simulink library "halin"  (R2021b)
settings: Solver=VariableStepAuto  StartTime=0.0  StopTime=10.0  RelTol=1e-3
undefined symbols (not defined in the file): TRUE
libraries: FVT_lib x177, hcu_lib x55
(part 8 of 17)

== system halin/HAL_IN/CAN3/BMS3 ==
  DT_CAN3_SG_BMS3 : Inport
  ACChrgCurrDis : Subsystem
  FireDetErr : Subsystem
  HVBChrgPwr : Subsystem
  HVBChrgPwrTotal : Subsystem
  HVBDrvPwr : Subsystem
  HVBDrvPwrTotal : Subsystem
  HVBFullChrgPwr : Subsystem
  HVBIsoImpedenceN : Subsystem
  HVBIsoImpedenceP : Subsystem
  HVBSOH : Subsystem
  HVBattErr : Subsystem
  HVBattPackVolt : Subsystem
  HVBattSOC : Subsystem
  HVBattSOCDis : Subsystem
  RemainChrgTime : Subsystem
  bus_selector : BusSelector  OutputSignals=CAN3_ACChrgCurrDis
  bus_selector1 : BusSelector  OutputSignals=CAN3_FireDetErr
  bus_selector10 : BusSelector  OutputSignals=CAN3_HVBattErr
  bus_selector11 : BusSelector  OutputSignals=CAN3_HVBattPackVolt
  bus_selector12 : BusSelector  OutputSignals=CAN3_HVBattSOC
  bus_selector13 : BusSelector  OutputSignals=CAN3_HVBattSOCDis
  bus_selector14 : BusSelector  OutputSignals=CAN3_RemainChrgTime
  bus_selector2 : BusSelector  OutputSignals=CAN3_HVBChrgPwr
  bus_selector3 : BusSelector  OutputSignals=CAN3_HVBChrgPwrTotal
  bus_selector4 : BusSelector  OutputSignals=CAN3_HVBDrvPwr
  bus_selector5 : BusSelector  OutputSignals=CAN3_HVBDrvPwrTotal
  bus_selector6 : BusSelector  OutputSignals=CAN3_HVBFullChrgPwr
  bus_selector7 : BusSelector  OutputSignals=CAN3_HVBIsoImpedenceN
  bus_selector8 : BusSelector  OutputSignals=CAN3_HVBIsoImpedenceP
  bus_selector9 : BusSelector  OutputSignals=CAN3_HVBSOH
  VHAL_ACChrgCurrDis_A : Outport
  VHAL_FireDetErr_flg : Outport  Port=2
  VHAL_HVBChrgPwr_kWh : Outport  Port=3
  VHAL_HVBChrgPwrTotal_kWh : Outport  Port=4
  VHAL_HVBDrvPwr_kWh : Outport  Port=5
  VHAL_HVBDrvPwrTotal_kWh : Outport  Port=6
  VHAL_HVBFullChrgPwr_kWh : Outport  Port=7
  VHAL_HVBIsoImpedenceN_Megaohm : Outport  Port=8
  VHAL_HVBIsoImpedenceP_Megaohm : Outport  Port=9
  VHAL_HVBSOH_pct : Outport  Port=10
  VHAL_HVBattErr_flg : Outport  Port=11
  VHAL_HVBattPackVolt_V : Outport  Port=12
  VHAL_HVBattSOC_pct : Outport  Port=13
  VHAL_HVBattSOCDis_pct : Outport  Port=14
  VHAL_RemainChrgTime_min : Outport  Port=15
  wires:
  DT_CAN3_SG_BMS3/1 -> [DT_CAN3_SG_BMS3]
  [DT_CAN3_SG_BMS3] -> bus_selector/1
  bus_selector/1 -> ACChrgCurrDis/1(ACChrgCurrDis)  "<CAN3_ACChrgCurrDis>"
  ACChrgCurrDis/1(VHAL_ACChrgCurrDis_A) -> VHAL_ACChrgCurrDis_A/1
  [DT_CAN3_SG_BMS3] -> bus_selector1/1
  bus_selector1/1 -> FireDetErr/1(FireDetErr)  "<CAN3_FireDetErr>"
  FireDetErr/1(VHAL_FireDetErr_flg) -> VHAL_FireDetErr_flg/1
  [DT_CAN3_SG_BMS3] -> bus_selector2/1
  bus_selector2/1 -> HVBChrgPwr/1(HVBChrgPwr)  "<CAN3_HVBChrgPwr>"
  HVBChrgPwr/1(VHAL_HVBChrgPwr_kWh) -> VHAL_HVBChrgPwr_kWh/1
  [DT_CAN3_SG_BMS3] -> bus_selector3/1
  bus_selector3/1 -> HVBChrgPwrTotal/1(HVBChrgPwrTotal)  "<CAN3_HVBChrgPwrTotal>"
  HVBChrgPwrTotal/1(VHAL_HVBChrgPwrTotal_kWh) -> VHAL_HVBChrgPwrTotal_kWh/1
  [DT_CAN3_SG_BMS3] -> bus_selector4/1
  bus_selector4/1 -> HVBDrvPwr/1(HVBDrvPwr)  "<CAN3_HVBDrvPwr>"
  HVBDrvPwr/1(VHAL_HVBDrvPwr_kWh) -> VHAL_HVBDrvPwr_kWh/1
  [DT_CAN3_SG_BMS3] -> bus_selector5/1
  bus_selector5/1 -> HVBDrvPwrTotal/1(HVBDrvPwrTotal)  "<CAN3_HVBDrvPwrTotal>"
  HVBDrvPwrTotal/1(VHAL_HVBDrvPwrTotal_kWh) -> VHAL_HVBDrvPwrTotal_kWh/1
  [DT_CAN3_SG_BMS3] -> bus_selector6/1
  bus_selector6/1 -> HVBFullChrgPwr/1(HVBFullChrgPwr)  "<CAN3_HVBFullChrgPwr>"
  HVBFullChrgPwr/1(VHAL_HVBFullChrgPwr_kWh) -> VHAL_HVBFullChrgPwr_kWh/1
  [DT_CAN3_SG_BMS3] -> bus_selector7/1
  bus_selector7/1 -> HVBIsoImpedenceN/1(HVBIsoImpedenceN)  "<CAN3_HVBIsoImpedenceN>"
  HVBIsoImpedenceN/1(VHAL_HVBIsoImpedenceN_Megaohm) -> VHAL_HVBIsoImpedenceN_Megaohm/1
  [DT_CAN3_SG_BMS3] -> bus_selector8/1
  bus_selector8/1 -> HVBIsoImpedenceP/1(HVBIsoImpedenceP)  "<CAN3_HVBIsoImpedenceP>"
  HVBIsoImpedenceP/1(VHAL_HVBIsoImpedenceP_Megaohm) -> VHAL_HVBIsoImpedenceP_Megaohm/1
  [DT_CAN3_SG_BMS3] -> bus_selector9/1
  bus_selector9/1 -> HVBSOH/1(HVBSOH)  "<CAN3_HVBSOH>"
  HVBSOH/1(VHAL_HVBSOH_pct) -> VHAL_HVBSOH_pct/1
  [DT_CAN3_SG_BMS3] -> bus_selector10/1
  bus_selector10/1 -> HVBattErr/1(HVBattErr)  "<CAN3_HVBattErr>"
  HVBattErr/1(VHAL_HVBattErr_flg) -> VHAL_HVBattErr_flg/1
  [DT_CAN3_SG_BMS3] -> bus_selector11/1
  bus_selector11/1 -> HVBattPackVolt/1(HVBattPackVolt)  "<CAN3_HVBattPackVolt>"
  HVBattPackVolt/1(VHAL_HVBattPackVolt_V) -> VHAL_HVBattPackVolt_V/1
  [DT_CAN3_SG_BMS3] -> bus_selector12/1
  bus_selector12/1 -> HVBattSOC/1(HVBattSOC)  "<CAN3_HVBattSOC>"
  HVBattSOC/1(VHAL_HVBattSOC_pct) -> VHAL_HVBattSOC_pct/1
  [DT_CAN3_SG_BMS3] -> bus_selector13/1
  bus_selector13/1 -> HVBattSOCDis/1(HVBattSOCDis)  "<CAN3_HVBattSOCDis>"
  HVBattSOCDis/1(VHAL_HVBattSOCDis_pct) -> VHAL_HVBattSOCDis_pct/1
  [DT_CAN3_SG_BMS3] -> bus_selector14/1
  bus_selector14/1 -> RemainChrgTime/1(RemainChrgTime)  "<CAN3_RemainChrgTime>"
  RemainChrgTime/1(VHAL_RemainChrgTime_min) -> VHAL_RemainChrgTime_min/1

== system halin/HAL_IN/CAN3/BMS4 ==
  DT_CAN3_SG_BMS4 : Inport
  CellTempAvg : Subsystem
  HVBCellVoltMax : Subsystem
  HVBCellVoltMin : Subsystem
  HVBMTempMax : Subsystem
  HVBMTempMin : Subsystem
  MaxCellTempNum : Subsystem
  MaxCellVoltNum : Subsystem
  MinCellTempNum : Subsystem
  MinCellVoltNum : Subsystem
  bus_selector : BusSelector  OutputSignals=CAN3_CellTempAvg
  bus_selector1 : BusSelector  OutputSignals=CAN3_HVBCellVoltMax
  bus_selector2 : BusSelector  OutputSignals=CAN3_HVBCellVoltMin
  bus_selector3 : BusSelector  OutputSignals=CAN3_HVBMTempMax
  bus_selector4 : BusSelector  OutputSignals=CAN3_HVBMTempMin
  bus_selector5 : BusSelector  OutputSignals=CAN3_MaxCellTemp_Num
  bus_selector6 : BusSelector  OutputSignals=CAN3_MaxCellVolt_Num
  bus_selector7 : BusSelector  OutputSignals=CAN3_MinCellTemp_Num
  bus_selector8 : BusSelector  OutputSignals=CAN3_MinCellVolt_Num
  VHAL_CellTempAvg_C : Outport
  VHAL_HVBCellVoltMax_mV : Outport  Port=2
  VHAL_HVBCellVoltMin_mV : Outport  Port=3
  VHAL_HVBMTempMax_C : Outport  Port=4
  VHAL_HVBMTempMin_C : Outport  Port=5
  VHAL_MaxCellTempNum_enum : Outport  Port=6
  VHAL_MaxCellVoltNum_enum : Outport  Port=7
  VHAL_MinCellTempNum_enum : Outport  Port=8
  VHAL_MinCellVoltNum_enum : Outport  Port=9
  wires:
  DT_CAN3_SG_BMS4/1 -> [DT_CAN3_SG_BMS4]
  [DT_CAN3_SG_BMS4] -> bus_selector/1
  bus_selector/1 -> CellTempAvg/1(CellTempAvg)  "<CAN3_CellTempAvg>"
  CellTempAvg/1(VHAL_CellTempAvg_C) -> VHAL_CellTempAvg_C/1
  [DT_CAN3_SG_BMS4] -> bus_selector1/1
  bus_selector1/1 -> HVBCellVoltMax/1(HVBCellVoltMax)  "<CAN3_HVBCellVoltMax>"
  HVBCellVoltMax/1(VHAL_HVBCellVoltMax_mV) -> VHAL_HVBCellVoltMax_mV/1
  [DT_CAN3_SG_BMS4] -> bus_selector2/1
  bus_selector2/1 -> HVBCellVoltMin/1(HVBCellVoltMin)  "<CAN3_HVBCellVoltMin>"
  HVBCellVoltMin/1(VHAL_HVBCellVoltMin_mV) -> VHAL_HVBCellVoltMin_mV/1
  [DT_CAN3_SG_BMS4] -> bus_selector3/1
  bus_selector3/1 -> HVBMTempMax/1(HVBMTempMax)  "<CAN3_HVBMTempMax>"
  HVBMTempMax/1(VHAL_HVBMTempMax_C) -> VHAL_HVBMTempMax_C/1
  [DT_CAN3_SG_BMS4] -> bus_selector4/1
  bus_selector4/1 -> HVBMTempMin/1(HVBMTempMin)  "<CAN3_HVBMTempMin>"
  HVBMTempMin/1(VHAL_HVBMTempMin_C) -> VHAL_HVBMTempMin_C/1
  [DT_CAN3_SG_BMS4] -> bus_selector5/1
  bus_selector5/1 -> MaxCellTempNum/1(MaxCellTemp_Num)  "<CAN3_MaxCellTemp_Num>"
  MaxCellTempNum/1(VHAL_MaxCellTempNum_enum) -> VHAL_MaxCellTempNum_enum/1
  [DT_CAN3_SG_BMS4] -> bus_selector6/1
  bus_selector6/1 -> MaxCellVoltNum/1(MaxCellVolt_Num)  "<CAN3_MaxCellVolt_Num>"
  MaxCellVoltNum/1(VHAL_MaxCellVoltNum_enum) -> VHAL_MaxCellVoltNum_enum/1
  [DT_CAN3_SG_BMS4] -> bus_selector7/1
  bus_selector7/1 -> MinCellTempNum/1(MinCellTemp_Num)  "<CAN3_MinCellTemp_Num>"
  MinCellTempNum/1(VHAL_MinCellTempNum_enum) -> VHAL_MinCellTempNum_enum/1
  [DT_CAN3_SG_BMS4] -> bus_selector8/1
  bus_selector8/1 -> MinCellVoltNum/1(MinCellVolt_Num)  "<CAN3_MinCellVolt_Num>"
  MinCellVoltNum/1(VHAL_MinCellVoltNum_enum) -> VHAL_MinCellVoltNum_enum/1

== system halin/HAL_IN/CAN3/BMS5 ==
  DT_CAN3_SG_BMS5 : Inport
  HVInVolt : Subsystem
  LVBattDet12V : Subsystem
  OBCACCSLimit : Subsystem
  OBCDCCurLm : Subsystem
  OBCDCVoltLm : Subsystem
  bus_selector : BusSelector  OutputSignals=CAN3_HVInVolt
  bus_selector1 : BusSelector  OutputSignals=CAN3_LVBattDet12V
  bus_selector2 : BusSelector  OutputSignals=CAN3_OBCACCSLimit
  bus_selector3 : BusSelector  OutputSignals=CAN3_OBCDCCurLm
  bus_selector4 : BusSelector  OutputSignals=CAN3_OBCDCVoltLm
  VHAL_HVInVolt_V : Outport
  VHAL_LVBattDet12V_V : Outport  Port=2
  VHAL_OBCACCSLimit_A : Outport  Port=3
  VHAL_OBCDCCurLm_A : Outport  Port=4
  VHAL_OBCDCVoltLm_V : Outport  Port=5
  wires:
  DT_CAN3_SG_BMS5/1 -> [DT_CAN3_SG_BMS5]
  [DT_CAN3_SG_BMS5] -> bus_selector/1
  bus_selector/1 -> HVInVolt/1(HVInVolt)  "<CAN3_HVInVolt>"
  HVInVolt/1(VHAL_HVInVolt_V) -> VHAL_HVInVolt_V/1
  [DT_CAN3_SG_BMS5] -> bus_selector1/1
  bus_selector1/1 -> LVBattDet12V/1(LVBattDet12V)  "<CAN3_LVBattDet12V>"
  LVBattDet12V/1(VHAL_LVBattDet12V_V) -> VHAL_LVBattDet12V_V/1
  [DT_CAN3_SG_BMS5] -> bus_selector2/1
  bus_selector2/1 -> OBCACCSLimit/1(OBCACCSLimit)  "<CAN3_OBCACCSLimit>"
  OBCACCSLimit/1(VHAL_OBCACCSLimit_A) -> VHAL_OBCACCSLimit_A/1
  [DT_CAN3_SG_BMS5] -> bus_selector3/1
  bus_selector3/1 -> OBCDCCurLm/1(OBCDCCurLm)  "<CAN3_OBCDCCurLm>"
  OBCDCCurLm/1(VHAL_OBCDCCurLm_A) -> VHAL_OBCDCCurLm_A/1
  [DT_CAN3_SG_BMS5] -> bus_selector4/1
  bus_selector4/1 -> OBCDCVoltLm/1(OBCDCVoltLm)  "<CAN3_OBCDCVoltLm>"
  OBCDCVoltLm/1(VHAL_OBCDCVoltLm_V) -> VHAL_OBCDCVoltLm_V/1

== system halin/HAL_IN/CAN3/BMS6 ==
  DT_CAN3_SG_BMS6 : Inport
  BMSChckSum : Subsystem
  BMSREADY : Subsystem
  BMSRolCnct : Subsystem
  BMSWarn1 : Subsystem
  BMSWarn2 : Subsystem
  BMSWarn3 : Subsystem
  BMSWarn4 : Subsystem
  BMSWarn5 : Subsystem
  BMSWarn6 : Subsystem
  BMSWarn7 : Subsystem
  BMSWarn8 : Subsystem
  ChrgInLockReq : Subsystem
  ChrgPlugSta : Subsystem
  DisChrgPlugErr : Subsystem
  ExtChrgSta : Subsystem
  HVBChrgErr : Subsystem
  HVBContactorSta : Subsystem
  HVBHVILErr : Subsystem
  HVBOvrTempErr : Subsystem
  HVBOvrTempWarn : Subsystem
  HVBPreheatPrecoolSta : Subsystem
  HVBattReady4Pre : Subsystem
  HVILSta : Subsystem
  V2LSta : Subsystem
  bus_selector : BusSelector  OutputSignals=CAN3_BMSChckSum
  bus_selector1 : BusSelector  OutputSignals=CAN3_BMSRolCnct
  bus_selector10 : BusSelector  OutputSignals=CAN3_BMS_Warn_8
  bus_selector11 : BusSelector  OutputSignals=CAN3_ChrgInLockReq
  bus_selector12 : BusSelector  OutputSignals=CAN3_ChrgPlugSta
  bus_selector13 : BusSelector  OutputSignals=CAN3_DisChrgPlugErr
  bus_selector14 : BusSelector  OutputSignals=CAN3_ExtChrgSta
  bus_selector15 : BusSelector  OutputSignals=CAN3_HVBChrgErr
  bus_selector16 : BusSelector  OutputSignals=CAN3_HVBContactorSta
  bus_selector17 : BusSelector  OutputSignals=CAN3_HVBHVILErr
  bus_selector18 : BusSelector  OutputSignals=CAN3_HVBOvrTempErr
  bus_selector19 : BusSelector  OutputSignals=CAN3_HVBOvrTempWarn
  bus_selector2 : BusSelector  OutputSignals=CAN3_BMS_READY
  bus_selector20 : BusSelector  OutputSignals=CAN3_HVBPreheatPrecoolSta
  bus_selector21 : BusSelector  OutputSignals=CAN3_HVBattReady4Pre
  bus_selector22 : BusSelector  OutputSignals=CAN3_HVILSta
  bus_selector23 : BusSelector  OutputSignals=CAN3_V2LSta
  bus_selector3 : BusSelector  OutputSignals=CAN3_BMS_Warn_1
  bus_selector4 : BusSelector  OutputSignals=CAN3_BMS_Warn_2
  bus_selector5 : BusSelector  OutputSignals=CAN3_BMS_Warn_3
  bus_selector6 : BusSelector  OutputSignals=CAN3_BMS_Warn_4
  bus_selector7 : BusSelector  OutputSignals=CAN3_BMS_Warn_5
  bus_selector8 : BusSelector  OutputSignals=CAN3_BMS_Warn_6
  bus_selector9 : BusSelector  OutputSignals=CAN3_BMS_Warn_7
  VHAL_BMSChckSum_enum : Outport
  VHAL_BMSRolCnct_enum : Outport  Port=2
  VHAL_BMSREADY_flg : Outport  Port=3
  VHAL_BMSWarn1_flg : Outport  Port=4
  VHAL_BMSWarn2_flg : Outport  Port=5
  VHAL_BMSWarn3_flg : Outport  Port=6
  VHAL_BMSWarn4_flg : Outport  Port=7
  VHAL_BMSWarn5_flg : Outport  Port=8
  VHAL_BMSWarn6_flg : Outport  Port=9
  VHAL_BMSWarn7_flg : Outport  Port=10
  VHAL_BMSWarn8_flg : Outport  Port=11
  VHAL_ChrgInLockReq_enum : Outport  Port=12
  VHAL_ChrgPlugSta_enum : Outport  Port=13
  VHAL_DisChrgPlugErr_enum : Outport  Port=14
  VHAL_ExtChrgSta_enum : Outport  Port=15
  VHAL_HVBChrgErr_enum : Outport  Port=16
  VHAL_HVBContactorSta_flg : Outport  Port=17
  VHAL_HVBHVILErr_flg : Outport  Port=18
  VHAL_HVBOvrTempErr_flg : Outport  Port=19
  VHAL_HVBOvrTempWarn_enum : Outport  Port=20
  VHAL_HVBPreheatPrecoolSta_enum : Outport  Port=21
  VHAL_HVBattReady4Pre_enum : Outport  Port=22
  VHAL_HVILSta_flg : Outport  Port=23
  VHAL_V2LSta_enum : Outport  Port=24
  wires:
  DT_CAN3_SG_BMS6/1 -> [DT_CAN3_SG_BMS6]
  [DT_CAN3_SG_BMS6] -> bus_selector/1
  bus_selector/1 -> BMSChckSum/1(BMSChckSum)  "<CAN3_BMSChckSum>"
  BMSChckSum/1(VHAL_BMSChckSum_enum) -> VHAL_BMSChckSum_enum/1
  [DT_CAN3_SG_BMS6] -> bus_selector1/1
  bus_selector1/1 -> BMSRolCnct/1(BMSRolCnct)  "<CAN3_BMSRolCnct>"
  BMSRolCnct/1(VHAL_BMSRolCnct_enum) -> VHAL_BMSRolCnct_enum/1
  [DT_CAN3_SG_BMS6] -> bus_selector2/1
  bus_selector2/1 -> BMSREADY/1(BMS_READY)  "<CAN3_BMS_READY>"
  BMSREADY/1(VHAL_BMSREADY_flg) -> VHAL_BMSREADY_flg/1
  [DT_CAN3_SG_BMS6] -> bus_selector3/1
  bus_selector3/1 -> BMSWarn1/1(BMS_Warn_1)  "<CAN3_BMS_Warn_1>"
  BMSWarn1/1(VHAL_BMSWarn1_flg) -> VHAL_BMSWarn1_flg/1
  [DT_CAN3_SG_BMS6] -> bus_selector4/1
  bus_selector4/1 -> BMSWarn2/1(BMS_Warn_2)  "<CAN3_BMS_Warn_2>"
  BMSWarn2/1(VHAL_BMSWarn2_flg) -> VHAL_BMSWarn2_flg/1
  [DT_CAN3_SG_BMS6] -> bus_selector5/1
  bus_selector5/1 -> BMSWarn3/1(BMS_Warn_3)  "<CAN3_BMS_Warn_3>"
  BMSWarn3/1(VHAL_BMSWarn3_flg) -> VHAL_BMSWarn3_flg/1
  [DT_CAN3_SG_BMS6] -> bus_selector6/1
  bus_selector6/1 -> BMSWarn4/1(BMS_Warn_4)  "<CAN3_BMS_Warn_4>"
  BMSWarn4/1(VHAL_BMSWarn4_flg) -> VHAL_BMSWarn4_flg/1
  [DT_CAN3_SG_BMS6] -> bus_selector7/1
  bus_selector7/1 -> BMSWarn5/1(BMS_Warn_5)  "<CAN3_BMS_Warn_5>"
  BMSWarn5/1(VHAL_BMSWarn5_flg) -> VHAL_BMSWarn5_flg/1
  [DT_CAN3_SG_BMS6] -> bus_selector8/1
  bus_selector8/1 -> BMSWarn6/1(BMS_Warn_6)  "<CAN3_BMS_Warn_6>"
  BMSWarn6/1(VHAL_BMSWarn6_flg) -> VHAL_BMSWarn6_flg/1
  [DT_CAN3_SG_BMS6] -> bus_selector9/1
  bus_selector9/1 -> BMSWarn7/1(BMS_Warn_7)  "<CAN3_BMS_Warn_7>"
  BMSWarn7/1(VHAL_BMSWarn7_flg) -> VHAL_BMSWarn7_flg/1
  [DT_CAN3_SG_BMS6] -> bus_selector10/1
  bus_selector10/1 -> BMSWarn8/1(BMS_Warn_8)  "<CAN3_BMS_Warn_8>"
  BMSWarn8/1(VHAL_BMSWarn8_flg) -> VHAL_BMSWarn8_flg/1
  [DT_CAN3_SG_BMS6] -> bus_selector11/1
  bus_selector11/1 -> ChrgInLockReq/1(ChrgInLockReq)  "<CAN3_ChrgInLockReq>"
  ChrgInLockReq/1(VHAL_ChrgInLockReq_enum) -> VHAL_ChrgInLockReq_enum/1
  [DT_CAN3_SG_BMS6] -> bus_selector12/1
  bus_selector12/1 -> ChrgPlugSta/1(ChrgPlugSta)  "<CAN3_ChrgPlugSta>"
  ChrgPlugSta/1(VHAL_ChrgPlugSta_enum) -> VHAL_ChrgPlugSta_enum/1
  [DT_CAN3_SG_BMS6] -> bus_selector13/1
  bus_selector13/1 -> DisChrgPlugErr/1(DisChrgPlugErr)  "<CAN3_DisChrgPlugErr>"
  DisChrgPlugErr/1(VHAL_DisChrgPlugErr_enum) -> VHAL_DisChrgPlugErr_enum/1
  [DT_CAN3_SG_BMS6] -> bus_selector14/1
  bus_selector14/1 -> ExtChrgSta/1(ExtChrgSta)  "<CAN3_ExtChrgSta>"
  ExtChrgSta/1(VHAL_ExtChrgSta_enum) -> VHAL_ExtChrgSta_enum/1
  [DT_CAN3_SG_BMS6] -> bus_selector15/1
  bus_selector15/1 -> HVBChrgErr/1(HVBChrgErr)  "<CAN3_HVBChrgErr>"
  HVBChrgErr/1(VHAL_HVBChrgErr_enum) -> VHAL_HVBChrgErr_enum/1
  [DT_CAN3_SG_BMS6] -> bus_selector16/1
  bus_selector16/1 -> HVBContactorSta/1(HVBContactorSta)  "<CAN3_HVBContactorSta>"
  HVBContactorSta/1(VHAL_HVBContactorSta_flg) -> VHAL_HVBContactorSta_flg/1
  [DT_CAN3_SG_BMS6] -> bus_selector17/1
  bus_selector17/1 -> HVBHVILErr/1(HVBHVILErr)  "<CAN3_HVBHVILErr>"
  HVBHVILErr/1(VHAL_HVBHVILErr_flg) -> VHAL_HVBHVILErr_flg/1
  [DT_CAN3_SG_BMS6] -> bus_selector18/1
  bus_selector18/1 -> HVBOvrTempErr/1(HVBOvrTempErr)  "<CAN3_HVBOvrTempErr>"
  HVBOvrTempErr/1(VHAL_HVBOvrTempErr_flg) -> VHAL_HVBOvrTempErr_flg/1
  [DT_CAN3_SG_BMS6] -> bus_selector19/1
  bus_selector19/1 -> HVBOvrTempWarn/1(HVBOvrTempWarn)  "<CAN3_HVBOvrTempWarn>"
  HVBOvrTempWarn/1(VHAL_HVBOvrTempWarn_enum) -> VHAL_HVBOvrTempWarn_enum/1
  [DT_CAN3_SG_BMS6] -> bus_selector20/1
  bus_selector20/1 -> HVBPreheatPrecoolSta/1(HVBPreheatPrecoolSta)  "<CAN3_HVBPreheatPrecoolSta>"
  HVBPreheatPrecoolSta/1(VHAL_HVBPreheatPrecoolSta_enum) -> VHAL_HVBPreheatPrecoolSta_enum/1
  [DT_CAN3_SG_BMS6] -> bus_selector21/1
  bus_selector21/1 -> HVBattReady4Pre/1(HVBattReady4Pre)  "<CAN3_HVBattReady4Pre>"
  HVBattReady4Pre/1(VHAL_HVBattReady4Pre_enum) -> VHAL_HVBattReady4Pre_enum/1
  [DT_CAN3_SG_BMS6] -> bus_selector22/1
  bus_selector22/1 -> HVILSta/1(HVILSta)  "<CAN3_HVILSta>"
  HVILSta/1(VHAL_HVILSta_flg) -> VHAL_HVILSta_flg/1
  [DT_CAN3_SG_BMS6] -> bus_selector23/1
  bus_selector23/1 -> V2LSta/1(V2LSta)  "<CAN3_V2LSta>"
  V2LSta/1(VHAL_V2LSta_enum) -> VHAL_V2LSta_enum/1

== system halin/HAL_IN/CAN3/BMS8 ==
  DT_CAN3_SG_BMS8 : Inport
  MainRlyNegSta : Subsystem
  MainRlyPosSta : Subsystem
  bus_selector : BusSelector  OutputSignals=CAN3_MainRlyNegSta
  bus_selector1 : BusSelector  OutputSignals=CAN3_MainRlyPosSta
  VHAL_MainRlyNegSta_enum : Outport
  VHAL_MainRlyPosSta_enum : Outport  Port=2
  wires:
  DT_CAN3_SG_BMS8/1 -> [DT_CAN3_SG_BMS8]
  [DT_CAN3_SG_BMS8] -> bus_selector/1
  bus_selector/1 -> MainRlyNegSta/1(MainRlyNegSta)  "<CAN3_MainRlyNegSta>"
  MainRlyNegSta/1(VHAL_MainRlyNegSta_enum) -> VHAL_MainRlyNegSta_enum/1
  [DT_CAN3_SG_BMS8] -> bus_selector1/1
  bus_selector1/1 -> MainRlyPosSta/1(MainRlyPosSta)  "<CAN3_MainRlyPosSta>"
  MainRlyPosSta/1(VHAL_MainRlyPosSta_enum) -> VHAL_MainRlyPosSta_enum/1

== system halin/HAL_IN/CAN3/CCU1 ==
  DT_CAN3_SG_CCU1 : Inport
  CSCCU1 : Subsystem
  DCDCAuxCur : Subsystem
  DCDCAuxVolt : Subsystem
  DCDCHVCur : Subsystem
  DCDCInVoltInf : Subsystem
  DCDCPreCompleted : Subsystem
  OBCDCCurrInf : Subsystem
  OBCDCVoltInf : Subsystem
  OBCPreCompleted : Subsystem
  OBCWakeup4Plugin : Subsystem
  RCCCU1 : Subsystem
  bus_selector : BusSelector  OutputSignals=CAN3_CS_CCU1
  bus_selector1 : BusSelector  OutputSignals=CAN3_DCDCAuxCur
  bus_selector10 : BusSelector  OutputSignals=CAN3_RC_CCU1
  bus_selector2 : BusSelector  OutputSignals=CAN3_DCDCAuxVolt
  bus_selector3 : BusSelector  OutputSignals=CAN3_DCDCHVCur
  bus_selector4 : BusSelector  OutputSignals=CAN3_DCDCInVoltInf
  bus_selector5 : BusSelector  OutputSignals=CAN3_DCDCPreCompleted
  bus_selector6 : BusSelector  OutputSignals=CAN3_OBCDCCurrInf
  bus_selector7 : BusSelector  OutputSignals=CAN3_OBCDCVoltInf
  bus_selector8 : BusSelector  OutputSignals=CAN3_OBCPreCompleted
  bus_selector9 : BusSelector  OutputSignals=CAN3_OBCWakeup4Plugin
  VHAL_CSCCU1_enum : Outport
  VHAL_DCDCAuxCur_A : Outport  Port=2
  VHAL_DCDCAuxVolt_V : Outport  Port=3
  VHAL_DCDCHVCur_A : Outport  Port=4
  VHAL_DCDCInVoltInf_V : Outport  Port=5
  VHAL_DCDCPreCompleted_enum : Outport  Port=6
  VHAL_OBCDCCurrInf_A : Outport  Port=7
  VHAL_OBCDCVoltInf_V : Outport  Port=8
  VHAL_OBCPreCompleted_enum : Outport  Port=9
  VHAL_OBCWakeup4Plugin_flg : Outport  Port=10
  VHAL_RCCCU1_enum : Outport  Port=11
  wires:
  DT_CAN3_SG_CCU1/1 -> [DT_CAN3_SG_CCU1]
  [DT_CAN3_SG_CCU1] -> bus_selector/1
  bus_selector/1 -> CSCCU1/1(CS_CCU1)  "<CAN3_CS_CCU1>"
  CSCCU1/1(VHAL_CSCCU1_enum) -> VHAL_CSCCU1_enum/1
  [DT_CAN3_SG_CCU1] -> bus_selector1/1
  bus_selector1/1 -> DCDCAuxCur/1(DCDCAuxCur)  "<CAN3_DCDCAuxCur>"
  DCDCAuxCur/1(VHAL_DCDCAuxCur_A) -> VHAL_DCDCAuxCur_A/1
  [DT_CAN3_SG_CCU1] -> bus_selector2/1
  bus_selector2/1 -> DCDCAuxVolt/1(DCDCAuxVolt)  "<CAN3_DCDCAuxVolt>"
  DCDCAuxVolt/1(VHAL_DCDCAuxVolt_V) -> VHAL_DCDCAuxVolt_V/1
  [DT_CAN3_SG_CCU1] -> bus_selector3/1
  bus_selector3/1 -> DCDCHVCur/1(DCDCHVCur)  "<CAN3_DCDCHVCur>"
  DCDCHVCur/1(VHAL_DCDCHVCur_A) -> VHAL_DCDCHVCur_A/1
  [DT_CAN3_SG_CCU1] -> bus_selector4/1
  bus_selector4/1 -> DCDCInVoltInf/1(DCDCInVoltInf)  "<CAN3_DCDCInVoltInf>"
  DCDCInVoltInf/1(VHAL_DCDCInVoltInf_V) -> VHAL_DCDCInVoltInf_V/1
  [DT_CAN3_SG_CCU1] -> bus_selector5/1
  bus_selector5/1 -> DCDCPreCompleted/1(DCDCPreCompleted)  "<CAN3_DCDCPreCompleted>"
  DCDCPreCompleted/1(VHAL_DCDCPreCompleted_enum) -> VHAL_DCDCPreCompleted_enum/1
  [DT_CAN3_SG_CCU1] -> bus_selector6/1
  bus_selector6/1 -> OBCDCCurrInf/1(OBCDCCurrInf)  "<CAN3_OBCDCCurrInf>"
  OBCDCCurrInf/1(VHAL_OBCDCCurrInf_A) -> VHAL_OBCDCCurrInf_A/1
  [DT_CAN3_SG_CCU1] -> bus_selector7/1
  bus_selector7/1 -> OBCDCVoltInf/1(OBCDCVoltInf)  "<CAN3_OBCDCVoltInf>"
  OBCDCVoltInf/1(VHAL_OBCDCVoltInf_V) -> VHAL_OBCDCVoltInf_V/1
  [DT_CAN3_SG_CCU1] -> bus_selector8/1
  bus_selector8/1 -> OBCPreCompleted/1(OBCPreCompleted)  "<CAN3_OBCPreCompleted>"
  OBCPreCompleted/1(VHAL_OBCPreCompleted_enum) -> VHAL_OBCPreCompleted_enum/1
  [DT_CAN3_SG_CCU1] -> bus_selector9/1
  bus_selector9/1 -> OBCWakeup4Plugin/1(OBCWakeup4Plugin)  "<CAN3_OBCWakeup4Plugin>"
  OBCWakeup4Plugin/1(VHAL_OBCWakeup4Plugin_flg) -> VHAL_OBCWakeup4Plugin_flg/1
  [DT_CAN3_SG_CCU1] -> bus_selector10/1
  bus_selector10/1 -> RCCCU1/1(RC_CCU1)  "<CAN3_RC_CCU1>"
  RCCCU1/1(VHAL_RCCCU1_enum) -> VHAL_RCCCU1_enum/1

== system halin/HAL_IN/CAN3/CCU2 ==
  DT_CAN3_SG_CCU2 : Inport
  CSCCU2 : Subsystem
  DCDCEnaSta : Subsystem
  DCDCFaultSta : Subsystem
  DCDCReady4Pre : Subsystem
  DCDCTemp : Subsystem
  OBCACCurLim : Subsystem
  OBCACCurrInf : Subsystem
  OBCACVoltInf : Subsystem
  OBCEnaSta : Subsystem
  OBCFaultSta : Subsystem
  OBCPluginSta : Subsystem
  OBCReady4Pre : Subsystem
  OBCTemp : Subsystem
  OBCV2LSta : Subsystem
  RCCCU2 : Subsystem
  bus_selector : BusSelector  OutputSignals=CAN3_CS_CCU2
  bus_selector1 : BusSelector  OutputSignals=CAN3_DCDCEnaSta
  bus_selector10 : BusSelector  OutputSignals=CAN3_OBCReady4Pre
  bus_selector11 : BusSelector  OutputSignals=CAN3_OBCTemp
  bus_selector12 : BusSelector  OutputSignals=CAN3_OBCV2LSta
  bus_selector13 : BusSelector  OutputSignals=CAN3_OBC_AC_Cur_Lim
  bus_selector14 : BusSelector  OutputSignals=CAN3_RC_CCU2
  bus_selector2 : BusSelector  OutputSignals=CAN3_DCDCFaultSta
  bus_selector3 : BusSelector  OutputSignals=CAN3_DCDCReady4Pre
  bus_selector4 : BusSelector  OutputSignals=CAN3_DCDCTemp
  bus_selector5 : BusSelector  OutputSignals=CAN3_OBCACCurrInf
  bus_selector6 : BusSelector  OutputSignals=CAN3_OBCACVoltInf
  bus_selector7 : BusSelector  OutputSignals=CAN3_OBCEnaSta
  bus_selector8 : BusSelector  OutputSignals=CAN3_OBCFaultSta
  bus_selector9 : BusSelector  OutputSignals=CAN3_OBCPluginSta
  VHAL_CSCCU2_enum : Outport
  VHAL_DCDCEnaSta_flg : Outport  Port=2
  VHAL_DCDCFaultSta_enum : Outport  Port=3
  VHAL_DCDCReady4Pre_flg : Outport  Port=4
  VHAL_DCDCTemp_C : Outport  Port=5
  VHAL_OBCACCurrInf_A : Outport  Port=6
  VHAL_OBCACVoltInf_V : Outport  Port=7
  VHAL_OBCEnaSta_flg : Outport  Port=8
  VHAL_OBCFaultSta_enum : Outport  Port=9
  VHAL_OBCPluginSta_flg : Outport  Port=10
  VHAL_OBCReady4Pre_flg : Outport  Port=11
  VHAL_OBCTemp_C : Outport  Port=12
  VHAL_OBCV2LSta_enum : Outport  Port=13
  VHAL_OBCACCurLim_enum : Outport  Port=14
  VHAL_RCCCU2_enum : Outport  Port=15
  wires:
  DT_CAN3_SG_CCU2/1 -> [DT_CAN3_SG_CCU2]
  [DT_CAN3_SG_CCU2] -> bus_selector/1
  bus_selector/1 -> CSCCU2/1(CS_CCU2)  "<CAN3_CS_CCU2>"
  CSCCU2/1(VHAL_CSCCU2_enum) -> VHAL_CSCCU2_enum/1
  [DT_CAN3_SG_CCU2] -> bus_selector1/1
  bus_selector1/1 -> DCDCEnaSta/1(DCDCEnaSta)  "<CAN3_DCDCEnaSta>"
  DCDCEnaSta/1(VHAL_DCDCEnaSta_flg) -> VHAL_DCDCEnaSta_flg/1
  [DT_CAN3_SG_CCU2] -> bus_selector2/1
  bus_selector2/1 -> DCDCFaultSta/1(DCDCFaultSta)  "<CAN3_DCDCFaultSta>"
  DCDCFaultSta/1(VHAL_DCDCFaultSta_enum) -> VHAL_DCDCFaultSta_enum/1
  [DT_CAN3_SG_CCU2] -> bus_selector3/1
  bus_selector3/1 -> DCDCReady4Pre/1(DCDCReady4Pre)  "<CAN3_DCDCReady4Pre>"
  DCDCReady4Pre/1(VHAL_DCDCReady4Pre_flg) -> VHAL_DCDCReady4Pre_flg/1
  [DT_CAN3_SG_CCU2] -> bus_selector4/1
  bus_selector4/1 -> DCDCTemp/1(DCDCTemp)  "<CAN3_DCDCTemp>"
  DCDCTemp/1(VHAL_DCDCTemp_C) -> VHAL_DCDCTemp_C/1
  [DT_CAN3_SG_CCU2] -> bus_selector5/1
  bus_selector5/1 -> OBCACCurrInf/1(OBCACCurrInf)  "<CAN3_OBCACCurrInf>"
  OBCACCurrInf/1(VHAL_OBCACCurrInf_A) -> VHAL_OBCACCurrInf_A/1
  [DT_CAN3_SG_CCU2] -> bus_selector6/1
  bus_selector6/1 -> OBCACVoltInf/1(OBCACVoltInf)  "<CAN3_OBCACVoltInf>"
  OBCACVoltInf/1(VHAL_OBCACVoltInf_V) -> VHAL_OBCACVoltInf_V/1
  [DT_CAN3_SG_CCU2] -> bus_selector7/1
  bus_selector7/1 -> OBCEnaSta/1(OBCEnaSta)  "<CAN3_OBCEnaSta>"
  OBCEnaSta/1(VHAL_OBCEnaSta_flg) -> VHAL_OBCEnaSta_flg/1
  [DT_CAN3_SG_CCU2] -> bus_selector8/1
  bus_selector8/1 -> OBCFaultSta/1(OBCFaultSta)  "<CAN3_OBCFaultSta>"
  OBCFaultSta/1(VHAL_OBCFaultSta_enum) -> VHAL_OBCFaultSta_enum/1
  [DT_CAN3_SG_CCU2] -> bus_selector9/1
  bus_selector9/1 -> OBCPluginSta/1(OBCPluginSta)  "<CAN3_OBCPluginSta>"
  OBCPluginSta/1(VHAL_OBCPluginSta_flg) -> VHAL_OBCPluginSta_flg/1
  [DT_CAN3_SG_CCU2] -> bus_selector10/1
  bus_selector10/1 -> OBCReady4Pre/1(OBCReady4Pre)  "<CAN3_OBCReady4Pre>"
  OBCReady4Pre/1(VHAL_OBCReady4Pre_flg) -> VHAL_OBCReady4Pre_flg/1
  [DT_CAN3_SG_CCU2] -> bus_selector11/1
  bus_selector11/1 -> OBCTemp/1(OBCTemp)  "<CAN3_OBCTemp>"
  OBCTemp/1(VHAL_OBCTemp_C) -> VHAL_OBCTemp_C/1
  [DT_CAN3_SG_CCU2] -> bus_selector12/1
  bus_selector12/1 -> OBCV2LSta/1(OBCV2LSta)  "<CAN3_OBCV2LSta>"
  OBCV2LSta/1(VHAL_OBCV2LSta_enum) -> VHAL_OBCV2LSta_enum/1
  [DT_CAN3_SG_CCU2] -> bus_selector13/1
  bus_selector13/1 -> OBCACCurLim/1(OBC_AC_Cur_Lim)  "<CAN3_OBC_AC_Cur_Lim>"
  OBCACCurLim/1(VHAL_OBCACCurLim_enum) -> VHAL_OBCACCurLim_enum/1
  [DT_CAN3_SG_CCU2] -> bus_selector14/1
  bus_selector14/1 -> RCCCU2/1(RC_CCU2)  "<CAN3_RC_CCU2>"
  RCCCU2/1(VHAL_RCCCU2_enum) -> VHAL_RCCCU2_enum/1

== system halin/HAL_IN/CAN3/EBM1 ==
  DT_CAN3_SG_EBM1 : Inport
  EBMErrSta : Subsystem
  EBMRLampSta : Subsystem
  bus_selector : BusSelector  OutputSignals=CAN3_EBMErrSta
  bus_selector1 : BusSelector  OutputSignals=CAN3_EBMRLampSta
  VHAL_EBMErrSta_enum : Outport
  VHAL_EBMRLampSta_enum : Outport  Port=2
  wires:
  DT_CAN3_SG_EBM1/1 -> [DT_CAN3_SG_EBM1]
  [DT_CAN3_SG_EBM1] -> bus_selector/1
  bus_selector/1 -> EBMErrSta/1(EBMErrSta)  "<CAN3_EBMErrSta>"
  EBMErrSta/1(VHAL_EBMErrSta_enum) -> VHAL_EBMErrSta_enum/1
  [DT_CAN3_SG_EBM1] -> bus_selector1/1
  bus_selector1/1 -> EBMRLampSta/1(EBMRLampSta)  "<CAN3_EBMRLampSta>"
  EBMRLampSta/1(VHAL_EBMRLampSta_enum) -> VHAL_EBMRLampSta_enum/1

== system halin/HAL_IN/CAN3/MCU_B_F1 ==
  DT_CAN3_SG_MCU_B_F1 : Inport
  FrActvDmpDisabSta : Subsystem
  FrEDUDrtSta : Subsystem
  FrEDUOpratingSta : Subsystem
  FrEDURealTMTq : Subsystem
  FrEDURotateDirction : Subsystem
  FrEDUTqReqFbk : Subsystem
  FrMCUBAT : Subsystem
  FrMCUDCBusCurr : Subsystem
  FrMCUDCBusVolt : Subsystem
  FrMCUDischrgSta : Subsystem
  FrMCUEnaSta : Subsystem
  FrMCUErr : Subsystem
  FrMCUIGNsta : Subsystem
  FrMCUReady : Subsystem
  FrMCUReady4Pre : Subsystem
  FrMCUSysSta : Subsystem
  FrMCUTemp : Subsystem
  FrMotorAvailTq : Subsystem
  FrRegenAvailTq : Subsystem
  FrTMSpd : Subsystem
  FrTMTemp : Subsystem
  FrTMid : Subsystem
  FrTMiq : Subsystem
  MCUWarnF : Subsystem
  bus_selector : BusSelector  OutputSignals=CAN3_Fr_ActvDmpDisabSta
  bus_selector1 : BusSelector  OutputSignals=CAN3_Fr_EDUDrtSta
  bus_selector10 : BusSelector  OutputSignals=CAN3_Fr_MCUEnaSta
  bus_selector11 : BusSelector  OutputSignals=CAN3_Fr_MCUErr
  bus_selector12 : BusSelector  OutputSignals=CAN3_Fr_MCUIGN_sta
  bus_selector13 : BusSelector  OutputSignals=CAN3_Fr_MCUReady
  bus_selector14 : BusSelector  OutputSignals=CAN3_Fr_MCUReady4Pre
  bus_selector15 : BusSelector  OutputSignals=CAN3_Fr_MCUSysSta
  bus_selector16 : BusSelector  OutputSignals=CAN3_Fr_MCUTemp
  bus_selector17 : BusSelector  OutputSignals=CAN3_Fr_MotorAvailTq
  bus_selector18 : BusSelector  OutputSignals=CAN3_Fr_RegenAvailTq
  bus_selector19 : BusSelector  OutputSignals=CAN3_Fr_TMSpd
  bus_selector2 : BusSelector  OutputSignals=CAN3_Fr_EDUOpratingSta
  bus_selector20 : BusSelector  OutputSignals=CAN3_Fr_TMTemp
  bus_selector21 : BusSelector  OutputSignals=CAN3_Fr_TMid
  bus_selector22 : BusSelector  OutputSignals=CAN3_Fr_TMiq
  bus_selector23 : BusSelector  OutputSignals=CAN3_MCUWarn_F
  bus_selector3 : BusSelector  OutputSignals=CAN3_Fr_EDURealTMTq
  bus_selector4 : BusSelector  OutputSignals=CAN3_Fr_EDURotateDirction
  bus_selector5 : BusSelector  OutputSignals=CAN3_Fr_EDUTqReqFbk
  bus_selector6 : BusSelector  OutputSignals=CAN3_Fr_MCUBAT
  bus_selector7 : BusSelector  OutputSignals=CAN3_Fr_MCUDCBusCurr
  bus_selector8 : BusSelector  OutputSignals=CAN3_Fr_MCUDCBusVolt
  bus_selector9 : BusSelector  OutputSignals=CAN3_Fr_MCUDischrgSta
  VHAL_FrActvDmpDisabSta_flg : Outport
  VHAL_FrEDUDrtSta_flg : Outport  Port=2
  VHAL_FrEDUOpratingSta_flg : Outport  Port=3
  VHAL_FrEDURealTMTq_Nm : Outport  Port=4
  VHAL_FrEDURotateDirction_enum : Outport  Port=5
  VHAL_FrEDUTqReqFbk_Nm : Outport  Port=6
  VHAL_FrMCUBAT_V : Outport  Port=7
  VHAL_FrMCUDCBusCurr_A : Outport  Port=8
  VHAL_FrMCUDCBusVolt_V : Outport  Port=9
  VHAL_FrMCUDischrgSta_flg : Outport  Port=10
  VHAL_FrMCUEnaSta_flg : Outport  Port=11
  VHAL_FrMCUErr_enum : Outport  Port=12
  VHAL_FrMCUIGNsta_flg : Outport  Port=13
  VHAL_FrMCUReady_flg : Outport  Port=14
  VHAL_FrMCUReady4Pre_flg : Outport  Port=15
  VHAL_FrMCUSysSta_enum : Outport  Port=16
  VHAL_FrMCUTemp_C : Outport  Port=17
  VHAL_FrMotorAvailTq_Nm : Outport  Port=18
  VHAL_FrRegenAvailTq_Nm : Outport  Port=19
  VHAL_FrTMSpd_rpm : Outport  Port=20
  VHAL_FrTMTemp_C : Outport  Port=21
  VHAL_FrTMid_A : Outport  Port=22
  VHAL_FrTMiq_A : Outport  Port=23
  VHAL_MCUWarnF_enum : Outport  Port=24
  wires:
  DT_CAN3_SG_MCU_B_F1/1 -> [DT_CAN3_SG_MCU_B_F1]
  [DT_CAN3_SG_MCU_B_F1] -> bus_selector/1
  bus_selector/1 -> FrActvDmpDisabSta/1(Fr_ActvDmpDisabSta)  "<CAN3_Fr_ActvDmpDisabSta>"
  FrActvDmpDisabSta/1(VHAL_FrActvDmpDisabSta_flg) -> VHAL_FrActvDmpDisabSta_flg/1
  [DT_CAN3_SG_MCU_B_F1] -> bus_selector1/1
  bus_selector1/1 -> FrEDUDrtSta/1(Fr_EDUDrtSta)  "<CAN3_Fr_EDUDrtSta>"
  FrEDUDrtSta/1(VHAL_FrEDUDrtSta_flg) -> VHAL_FrEDUDrtSta_flg/1
  [DT_CAN3_SG_MCU_B_F1] -> bus_selector2/1
  bus_selector2/1 -> FrEDUOpratingSta/1(Fr_EDUOpratingSta)  "<CAN3_Fr_EDUOpratingSta>"
  FrEDUOpratingSta/1(VHAL_FrEDUOpratingSta_flg) -> VHAL_FrEDUOpratingSta_flg/1
  [DT_CAN3_SG_MCU_B_F1] -> bus_selector3/1
  bus_selector3/1 -> FrEDURealTMTq/1(Fr_EDURealTMTq)  "<CAN3_Fr_EDURealTMTq>"
  FrEDURealTMTq/1(VHAL_FrEDURealTMTq_Nm) -> VHAL_FrEDURealTMTq_Nm/1
  [DT_CAN3_SG_MCU_B_F1] -> bus_selector4/1
  bus_selector4/1 -> FrEDURotateDirction/1(Fr_EDURotateDirction)  "<CAN3_Fr_EDURotateDirction>"
  FrEDURotateDirction/1(VHAL_FrEDURotateDirction_enum) -> VHAL_FrEDURotateDirction_enum/1
  [DT_CAN3_SG_MCU_B_F1] -> bus_selector5/1
  bus_selector5/1 -> FrEDUTqReqFbk/1(Fr_EDUTqReqFbk)  "<CAN3_Fr_EDUTqReqFbk>"
  FrEDUTqReqFbk/1(VHAL_FrEDUTqReqFbk_Nm) -> VHAL_FrEDUTqReqFbk_Nm/1
  [DT_CAN3_SG_MCU_B_F1] -> bus_selector6/1
  bus_selector6/1 -> FrMCUBAT/1(Fr_MCUBAT)  "<CAN3_Fr_MCUBAT>"
  FrMCUBAT/1(VHAL_FrMCUBAT_V) -> VHAL_FrMCUBAT_V/1
  [DT_CAN3_SG_MCU_B_F1] -> bus_selector7/1
  bus_selector7/1 -> FrMCUDCBusCurr/1(Fr_MCUDCBusCurr)  "<CAN3_Fr_MCUDCBusCurr>"
  FrMCUDCBusCurr/1(VHAL_FrMCUDCBusCurr_A) -> VHAL_FrMCUDCBusCurr_A/1
  [DT_CAN3_SG_MCU_B_F1] -> bus_selector8/1
  bus_selector8/1 -> FrMCUDCBusVolt/1(Fr_MCUDCBusVolt)  "<CAN3_Fr_MCUDCBusVolt>"
  FrMCUDCBusVolt/1(VHAL_FrMCUDCBusVolt_V) -> VHAL_FrMCUDCBusVolt_V/1
  [DT_CAN3_SG_MCU_B_F1] -> bus_selector9/1
  bus_selector9/1 -> FrMCUDischrgSta/1(Fr_MCUDischrgSta)  "<CAN3_Fr_MCUDischrgSta>"
  FrMCUDischrgSta/1(VHAL_FrMCUDischrgSta_flg) -> VHAL_FrMCUDischrgSta_flg/1
  [DT_CAN3_SG_MCU_B_F1] -> bus_selector10/1
  bus_selector10/1 -> FrMCUEnaSta/1(Fr_MCUEnaSta)  "<CAN3_Fr_MCUEnaSta>"
  FrMCUEnaSta/1(VHAL_FrMCUEnaSta_flg) -> VHAL_FrMCUEnaSta_flg/1
  [DT_CAN3_SG_MCU_B_F1] -> bus_selector11/1
  bus_selector11/1 -> FrMCUErr/1(Fr_MCUErr)  "<CAN3_Fr_MCUErr>"
  FrMCUErr/1(VHAL_FrMCUErr_enum) -> VHAL_FrMCUErr_enum/1
  [DT_CAN3_SG_MCU_B_F1] -> bus_selector12/1
  bus_selector12/1 -> FrMCUIGNsta/1(Fr_MCUIGN_sta)  "<CAN3_Fr_MCUIGN_sta>"
  FrMCUIGNsta/1(VHAL_FrMCUIGNsta_flg) -> VHAL_FrMCUIGNsta_flg/1
  [DT_CAN3_SG_MCU_B_F1] -> bus_selector13/1
  bus_selector13/1 -> FrMCUReady/1(Fr_MCUReady)  "<CAN3_Fr_MCUReady>"
  FrMCUReady/1(VHAL_FrMCUReady_flg) -> VHAL_FrMCUReady_flg/1
  [DT_CAN3_SG_MCU_B_F1] -> bus_selector14/1
  bus_selector14/1 -> FrMCUReady4Pre/1(Fr_MCUReady4Pre)  "<CAN3_Fr_MCUReady4Pre>"
  FrMCUReady4Pre/1(VHAL_FrMCUReady4Pre_flg) -> VHAL_FrMCUReady4Pre_flg/1
  [DT_CAN3_SG_MCU_B_F1] -> bus_selector15/1
  bus_selector15/1 -> FrMCUSysSta/1(Fr_MCUSysSta)  "<CAN3_Fr_MCUSysSta>"
  FrMCUSysSta/1(VHAL_FrMCUSysSta_enum) -> VHAL_FrMCUSysSta_enum/1
  [DT_CAN3_SG_MCU_B_F1] -> bus_selector16/1
  bus_selector16/1 -> FrMCUTemp/1(Fr_MCUTemp)  "<CAN3_Fr_MCUTemp>"
  FrMCUTemp/1(VHAL_FrMCUTemp_C) -> VHAL_FrMCUTemp_C/1
  [DT_CAN3_SG_MCU_B_F1] -> bus_selector17/1
  bus_selector17/1 -> FrMotorAvailTq/1(Fr_MotorAvailTq)  "<CAN3_Fr_MotorAvailTq>"
  FrMotorAvailTq/1(VHAL_FrMotorAvailTq_Nm) -> VHAL_FrMotorAvailTq_Nm/1
  [DT_CAN3_SG_MCU_B_F1] -> bus_selector18/1
  bus_selector18/1 -> FrRegenAvailTq/1(Fr_RegenAvailTq)  "<CAN3_Fr_RegenAvailTq>"
  FrRegenAvailTq/1(VHAL_FrRegenAvailTq_Nm) -> VHAL_FrRegenAvailTq_Nm/1
  [DT_CAN3_SG_MCU_B_F1] -> bus_selector19/1
  bus_selector19/1 -> FrTMSpd/1(Fr_TMSpd)  "<CAN3_Fr_TMSpd>"
  FrTMSpd/1(VHAL_FrTMSpd_rpm) -> VHAL_FrTMSpd_rpm/1
  [DT_CAN3_SG_MCU_B_F1] -> bus_selector20/1
  bus_selector20/1 -> FrTMTemp/1(Fr_TMTemp)  "<CAN3_Fr_TMTemp>"
  FrTMTemp/1(VHAL_FrTMTemp_C) -> VHAL_FrTMTemp_C/1
  [DT_CAN3_SG_MCU_B_F1] -> bus_selector21/1
  bus_selector21/1 -> FrTMid/1(Fr_TMid)  "<CAN3_Fr_TMid>"
  FrTMid/1(VHAL_FrTMid_A) -> VHAL_FrTMid_A/1
  [DT_CAN3_SG_MCU_B_F1] -> bus_selector22/1
  bus_selector22/1 -> FrTMiq/1(Fr_TMiq)  "<CAN3_Fr_TMiq>"
  FrTMiq/1(VHAL_FrTMiq_A) -> VHAL_FrTMiq_A/1
  [DT_CAN3_SG_MCU_B_F1] -> bus_selector23/1
  bus_selector23/1 -> MCUWarnF/1(MCUWarn_F)  "<CAN3_MCUWarn_F>"
  MCUWarnF/1(VHAL_MCUWarnF_enum) -> VHAL_MCUWarnF_enum/1

== system halin/HAL_IN/CAN3/MCU_B_F2 ==
  DT_CAN3_SG_MCU_B_F2 : Inport
  FrCoolanttempReq : Subsystem
  FrFailcode1 : Subsystem
  FrFailcode2 : Subsystem
  FrFailcodehistory1 : Subsystem
  FrFailcodehistory2 : Subsystem
  FrLLCTemp : Subsystem
  FrLLCflowReq : Subsystem
  FrMCUHWVer : Subsystem
  FrMCUSWVer : Subsystem
  FrMCUTempWarn : Subsystem
  FrTMTempWarn : Subsystem
  MCUBFLLCTempWarnSta : Subsystem
  bus_selector : BusSelector  OutputSignals=CAN3_Fr_CoolanttempReq
  bus_selector1 : BusSelector  OutputSignals=CAN3_Fr_Failcode1
  bus_selector10 : BusSelector  OutputSignals=CAN3_Fr_TMTempWarn
  bus_selector11 : BusSelector  OutputSignals=CAN3_MCU_B_F_LLCTempWarn_Sta
  bus_selector2 : BusSelector  OutputSignals=CAN3_Fr_Failcode2
  bus_selector3 : BusSelector  OutputSignals=CAN3_Fr_Failcodehistory1
  bus_selector4 : BusSelector  OutputSignals=CAN3_Fr_Failcodehistory2
  bus_selector5 : BusSelector  OutputSignals=CAN3_Fr_LLCTemp
  bus_selector6 : BusSelector  OutputSignals=CAN3_Fr_LLCflowReq
  bus_selector7 : BusSelector  OutputSignals=CAN3_Fr_MCUTempWarn
  bus_selector8 : BusSelector  OutputSignals=CAN3_Fr_MCU_HW_Ver
  bus_selector9 : BusSelector  OutputSignals=CAN3_Fr_MCU_SW_Ver
  VHAL_FrCoolanttempReq_C : Outport
  VHAL_FrFailcode1_enum : Outport  Port=2
  VHAL_FrFailcode2_enum : Outport  Port=3
  VHAL_FrFailcodehistory1_enum : Outport  Port=4
  VHAL_FrFailcodehistory2_enum : Outport  Port=5
  VHAL_FrLLCTemp_C : Outport  Port=6
  VHAL_FrLLCflowReq_Lpmin : Outport  Port=7
  VHAL_FrMCUTempWarn_enum : Outport  Port=8
  VHAL_FrMCUHWVer_enum : Outport  Port=9
  VHAL_FrMCUSWVer_enum : Outport  Port=10
  VHAL_FrTMTempWarn_enum : Outport  Port=11
  VHAL_MCUBFLLCTempWarnSta_enum : Outport  Port=12
  wires:
  DT_CAN3_SG_MCU_B_F2/1 -> [DT_CAN3_SG_MCU_B_F2]
  [DT_CAN3_SG_MCU_B_F2] -> bus_selector/1
  bus_selector/1 -> FrCoolanttempReq/1(Fr_CoolanttempReq)  "<CAN3_Fr_CoolanttempReq>"
  FrCoolanttempReq/1(VHAL_FrCoolanttempReq_C) -> VHAL_FrCoolanttempReq_C/1
  [DT_CAN3_SG_MCU_B_F2] -> bus_selector1/1
  bus_selector1/1 -> FrFailcode1/1(Fr_Failcode1)  "<CAN3_Fr_Failcode1>"
  FrFailcode1/1(VHAL_FrFailcode1_enum) -> VHAL_FrFailcode1_enum/1
  [DT_CAN3_SG_MCU_B_F2] -> bus_selector2/1
  bus_selector2/1 -> FrFailcode2/1(Fr_Failcode2)  "<CAN3_Fr_Failcode2>"
  FrFailcode2/1(VHAL_FrFailcode2_enum) -> VHAL_FrFailcode2_enum/1
  [DT_CAN3_SG_MCU_B_F2] -> bus_selector3/1
  bus_selector3/1 -> FrFailcodehistory1/1(Fr_Failcodehistory1)  "<CAN3_Fr_Failcodehistory1>"
  FrFailcodehistory1/1(VHAL_FrFailcodehistory1_enum) -> VHAL_FrFailcodehistory1_enum/1
  [DT_CAN3_SG_MCU_B_F2] -> bus_selector4/1
  bus_selector4/1 -> FrFailcodehistory2/1(Fr_Failcodehistory2)  "<CAN3_Fr_Failcodehistory2>"
  FrFailcodehistory2/1(VHAL_FrFailcodehistory2_enum) -> VHAL_FrFailcodehistory2_enum/1
  [DT_CAN3_SG_MCU_B_F2] -> bus_selector5/1
  bus_selector5/1 -> FrLLCTemp/1(Fr_LLCTemp)  "<CAN3_Fr_LLCTemp>"
  FrLLCTemp/1(VHAL_FrLLCTemp_C) -> VHAL_FrLLCTemp_C/1
  [DT_CAN3_SG_MCU_B_F2] -> bus_selector6/1
  bus_selector6/1 -> FrLLCflowReq/1(Fr_LLCflowReq)  "<CAN3_Fr_LLCflowReq>"
  FrLLCflowReq/1(VHAL_FrLLCflowReq_Lpmin) -> VHAL_FrLLCflowReq_Lpmin/1
  [DT_CAN3_SG_MCU_B_F2] -> bus_selector7/1
  bus_selector7/1 -> FrMCUTempWarn/1(Fr_MCUTempWarn)  "<CAN3_Fr_MCUTempWarn>"
  FrMCUTempWarn/1(VHAL_FrMCUTempWarn_enum) -> VHAL_FrMCUTempWarn_enum/1
  [DT_CAN3_SG_MCU_B_F2] -> bus_selector8/1
  bus_selector8/1 -> FrMCUHWVer/1(Fr_MCU_HW_Ver)  "<CAN3_Fr_MCU_HW_Ver>"
  FrMCUHWVer/1(VHAL_FrMCUHWVer_enum) -> VHAL_FrMCUHWVer_enum/1
  [DT_CAN3_SG_MCU_B_F2] -> bus_selector9/1
  bus_selector9/1 -> FrMCUSWVer/1(Fr_MCU_SW_Ver)  "<CAN3_Fr_MCU_SW_Ver>"
  FrMCUSWVer/1(VHAL_FrMCUSWVer_enum) -> VHAL_FrMCUSWVer_enum/1
  [DT_CAN3_SG_MCU_B_F2] -> bus_selector10/1
  bus_selector10/1 -> FrTMTempWarn/1(Fr_TMTempWarn)  "<CAN3_Fr_TMTempWarn>"
  FrTMTempWarn/1(VHAL_FrTMTempWarn_enum) -> VHAL_FrTMTempWarn_enum/1
  [DT_CAN3_SG_MCU_B_F2] -> bus_selector11/1
  bus_selector11/1 -> MCUBFLLCTempWarnSta/1(MCU_B_F_LLCTempWarn_Sta)  "<CAN3_MCU_B_F_LLCTempWarn_Sta>"
  MCUBFLLCTempWarnSta/1(VHAL_MCUBFLLCTempWarnSta_enum) -> VHAL_MCUBFLLCTempWarnSta_enum/1

== system halin/HAL_IN/CAN3/MCU_B_R1 ==
  DT_CAN3_SG_MCU_B_R1 : Inport
  MCUWarnR : Subsystem
  RrActvDmpDisabSta : Subsystem
  RrEDUDrtSta : Subsystem
  RrEDUOpratingSta : Subsystem
  RrEDURealTMTq : Subsystem
  RrEDURotateDirction : Subsystem
  RrEDUTqReqFbk : Subsystem
  RrMCUBAT : Subsystem
  RrMCUDCBusCurr : Subsystem
  RrMCUDCBusVolt : Subsystem
  RrMCUDischrgSta : Subsystem
  RrMCUEnaSta : Subsystem
  RrMCUErr : Subsystem
  RrMCUIGNsta : Subsystem
  RrMCUReady : Subsystem
  RrMCUReady4Pre : Subsystem
  RrMCUSysSta : Subsystem
  RrMCUTemp : Subsystem
  RrMotorAvailTq : Subsystem
  RrRegenAvailTq : Subsystem
  RrTMSpd : Subsystem
  RrTMTemp : Subsystem
  RrTMid : Subsystem
  RrTMiq : Subsystem
  bus_selector : BusSelector  OutputSignals=CAN3_MCUWarn_R
  bus_selector1 : BusSelector  OutputSignals=CAN3_Rr_ActvDmpDisabSta
  bus_selector10 : BusSelector  OutputSignals=CAN3_Rr_MCUDischrgSta
  bus_selector11 : BusSelector  OutputSignals=CAN3_Rr_MCUEnaSta
  bus_selector12 : BusSelector  OutputSignals=CAN3_Rr_MCUErr
  bus_selector13 : BusSelector  OutputSignals=CAN3_Rr_MCUIGN_sta
  bus_selector14 : BusSelector  OutputSignals=CAN3_Rr_MCUReady
  bus_selector15 : BusSelector  OutputSignals=CAN3_Rr_MCUReady4Pre
  bus_selector16 : BusSelector  OutputSignals=CAN3_Rr_MCUSysSta
  bus_selector17 : BusSelector  OutputSignals=CAN3_Rr_MCUTemp
  bus_selector18 : BusSelector  OutputSignals=CAN3_Rr_MotorAvailTq
  bus_selector19 : BusSelector  OutputSignals=CAN3_Rr_RegenAvailTq
  bus_selector2 : BusSelector  OutputSignals=CAN3_Rr_EDUDrtSta
  bus_selector20 : BusSelector  OutputSignals=CAN3_Rr_TMSpd
  bus_selector21 : BusSelector  OutputSignals=CAN3_Rr_TMTemp
  bus_selector22 : BusSelector  OutputSignals=CAN3_Rr_TMid
  bus_selector23 : BusSelector  OutputSignals=CAN3_Rr_TMiq
  bus_selector3 : BusSelector  OutputSignals=CAN3_Rr_EDUOpratingSta
  bus_selector4 : BusSelector  OutputSignals=CAN3_Rr_EDURealTMTq
  bus_selector5 : BusSelector  OutputSignals=CAN3_Rr_EDURotateDirction
  bus_selector6 : BusSelector  OutputSignals=CAN3_Rr_EDUTqReqFbk
  bus_selector7 : BusSelector  OutputSignals=CAN3_Rr_MCUBAT
  bus_selector8 : BusSelector  OutputSignals=CAN3_Rr_MCUDCBusCurr
  bus_selector9 : BusSelector  OutputSignals=CAN3_Rr_MCUDCBusVolt
  VHAL_MCUWarnR_enum : Outport
  VHAL_RrActvDmpDisabSta_flg : Outport  Port=2
  VHAL_RrEDUDrtSta_flg : Outport  Port=3
  VHAL_RrEDUOpratingSta_flg : Outport  Port=4
  VHAL_RrEDURealTMTq_Nm : Outport  Port=5
  VHAL_RrEDURotateDirction_enum : Outport  Port=6
  VHAL_RrEDUTqReqFbk_Nm : Outport  Port=7
  VHAL_RrMCUBAT_V : Outport  Port=8
  VHAL_RrMCUDCBusCurr_A : Outport  Port=9
  VHAL_RrMCUDCBusVolt_V : Outport  Port=10
  VHAL_RrMCUDischrgSta_flg : Outport  Port=11
  VHAL_RrMCUEnaSta_flg : Outport  Port=12
  VHAL_RrMCUErr_enum : Outport  Port=13
  VHAL_RrMCUIGNsta_flg : Outport  Port=14
  VHAL_RrMCUReady_flg : Outport  Port=15
  VHAL_RrMCUReady4Pre_flg : Outport  Port=16
  VHAL_RrMCUSysSta_enum : Outport  Port=17
  VHAL_RrMCUTemp_C : Outport  Port=18
  VHAL_RrMotorAvailTq_Nm : Outport  Port=19
  VHAL_RrRegenAvailTq_Nm : Outport  Port=20
  VHAL_RrTMSpd_rpm : Outport  Port=21
  VHAL_RrTMTemp_C : Outport  Port=22
  VHAL_RrTMid_A : Outport  Port=23
  VHAL_RrTMiq_A : Outport  Port=24
  wires:
  DT_CAN3_SG_MCU_B_R1/1 -> [DT_CAN3_SG_MCU_B_R1]
  [DT_CAN3_SG_MCU_B_R1] -> bus_selector/1
  bus_selector/1 -> MCUWarnR/1(MCUWarn_R)  "<CAN3_MCUWarn_R>"
  MCUWarnR/1(VHAL_MCUWarnR_enum) -> VHAL_MCUWarnR_enum/1
  [DT_CAN3_SG_MCU_B_R1] -> bus_selector1/1
  bus_selector1/1 -> RrActvDmpDisabSta/1(Rr_ActvDmpDisabSta)  "<CAN3_Rr_ActvDmpDisabSta>"
  RrActvDmpDisabSta/1(VHAL_RrActvDmpDisabSta_flg) -> VHAL_RrActvDmpDisabSta_flg/1
  [DT_CAN3_SG_MCU_B_R1] -> bus_selector2/1
  bus_selector2/1 -> RrEDUDrtSta/1(Rr_EDUDrtSta)  "<CAN3_Rr_EDUDrtSta>"
  RrEDUDrtSta/1(VHAL_RrEDUDrtSta_flg) -> VHAL_RrEDUDrtSta_flg/1
  [DT_CAN3_SG_MCU_B_R1] -> bus_selector3/1
  bus_selector3/1 -> RrEDUOpratingSta/1(Rr_EDUOpratingSta)  "<CAN3_Rr_EDUOpratingSta>"
  RrEDUOpratingSta/1(VHAL_RrEDUOpratingSta_flg) -> VHAL_RrEDUOpratingSta_flg/1
  [DT_CAN3_SG_MCU_B_R1] -> bus_selector4/1
  bus_selector4/1 -> RrEDURealTMTq/1(Rr_EDURealTMTq)  "<CAN3_Rr_EDURealTMTq>"
  RrEDURealTMTq/1(VHAL_RrEDURealTMTq_Nm) -> VHAL_RrEDURealTMTq_Nm/1
  [DT_CAN3_SG_MCU_B_R1] -> bus_selector5/1
  bus_selector5/1 -> RrEDURotateDirction/1(Rr_EDURotateDirction)  "<CAN3_Rr_EDURotateDirction>"
  RrEDURotateDirction/1(VHAL_RrEDURotateDirction_enum) -> VHAL_RrEDURotateDirction_enum/1
  [DT_CAN3_SG_MCU_B_R1] -> bus_selector6/1
  bus_selector6/1 -> RrEDUTqReqFbk/1(Rr_EDUTqReqFbk)  "<CAN3_Rr_EDUTqReqFbk>"
  RrEDUTqReqFbk/1(VHAL_RrEDUTqReqFbk_Nm) -> VHAL_RrEDUTqReqFbk_Nm/1
  [DT_CAN3_SG_MCU_B_R1] -> bus_selector7/1
  bus_selector7/1 -> RrMCUBAT/1(Rr_MCUBAT)  "<CAN3_Rr_MCUBAT>"
  RrMCUBAT/1(VHAL_RrMCUBAT_V) -> VHAL_RrMCUBAT_V/1
  [DT_CAN3_SG_MCU_B_R1] -> bus_selector8/1
  bus_selector8/1 -> RrMCUDCBusCurr/1(Rr_MCUDCBusCurr)  "<CAN3_Rr_MCUDCBusCurr>"
  RrMCUDCBusCurr/1(VHAL_RrMCUDCBusCurr_A) -> VHAL_RrMCUDCBusCurr_A/1
  [DT_CAN3_SG_MCU_B_R1] -> bus_selector9/1
  bus_selector9/1 -> RrMCUDCBusVolt/1(Rr_MCUDCBusVolt)  "<CAN3_Rr_MCUDCBusVolt>"
  RrMCUDCBusVolt/1(VHAL_RrMCUDCBusVolt_V) -> VHAL_RrMCUDCBusVolt_V/1
  [DT_CAN3_SG_MCU_B_R1] -> bus_selector10/1
  bus_selector10/1 -> RrMCUDischrgSta/1(Rr_MCUDischrgSta)  "<CAN3_Rr_MCUDischrgSta>"
  RrMCUDischrgSta/1(VHAL_RrMCUDischrgSta_flg) -> VHAL_RrMCUDischrgSta_flg/1
  [DT_CAN3_SG_MCU_B_R1] -> bus_selector11/1
  bus_selector11/1 -> RrMCUEnaSta/1(Rr_MCUEnaSta)  "<CAN3_Rr_MCUEnaSta>"
  RrMCUEnaSta/1(VHAL_RrMCUEnaSta_flg) -> VHAL_RrMCUEnaSta_flg/1
  [DT_CAN3_SG_MCU_B_R1] -> bus_selector12/1
  bus_selector12/1 -> RrMCUErr/1(Rr_MCUErr)  "<CAN3_Rr_MCUErr>"
  RrMCUErr/1(VHAL_RrMCUErr_enum) -> VHAL_RrMCUErr_enum/1
  [DT_CAN3_SG_MCU_B_R1] -> bus_selector13/1
  bus_selector13/1 -> RrMCUIGNsta/1(Rr_MCUIGN_sta)  "<CAN3_Rr_MCUIGN_sta>"
  RrMCUIGNsta/1(VHAL_RrMCUIGNsta_flg) -> VHAL_RrMCUIGNsta_flg/1
  [DT_CAN3_SG_MCU_B_R1] -> bus_selector14/1
  bus_selector14/1 -> RrMCUReady/1(Rr_MCUReady)  "<CAN3_Rr_MCUReady>"
  RrMCUReady/1(VHAL_RrMCUReady_flg) -> VHAL_RrMCUReady_flg/1
  [DT_CAN3_SG_MCU_B_R1] -> bus_selector15/1
  bus_selector15/1 -> RrMCUReady4Pre/1(Rr_MCUReady4Pre)  "<CAN3_Rr_MCUReady4Pre>"
  RrMCUReady4Pre/1(VHAL_RrMCUReady4Pre_flg) -> VHAL_RrMCUReady4Pre_flg/1
  [DT_CAN3_SG_MCU_B_R1] -> bus_selector16/1
  bus_selector16/1 -> RrMCUSysSta/1(Rr_MCUSysSta)  "<CAN3_Rr_MCUSysSta>"
  RrMCUSysSta/1(VHAL_RrMCUSysSta_enum) -> VHAL_RrMCUSysSta_enum/1
  [DT_CAN3_SG_MCU_B_R1] -> bus_selector17/1
  bus_selector17/1 -> RrMCUTemp/1(Rr_MCUTemp)  "<CAN3_Rr_MCUTemp>"
  RrMCUTemp/1(VHAL_RrMCUTemp_C) -> VHAL_RrMCUTemp_C/1
  [DT_CAN3_SG_MCU_B_R1] -> bus_selector18/1
  bus_selector18/1 -> RrMotorAvailTq/1(Rr_MotorAvailTq)  "<CAN3_Rr_MotorAvailTq>"
  RrMotorAvailTq/1(VHAL_RrMotorAvailTq_Nm) -> VHAL_RrMotorAvailTq_Nm/1
  [DT_CAN3_SG_MCU_B_R1] -> bus_selector19/1
  bus_selector19/1 -> RrRegenAvailTq/1(Rr_RegenAvailTq)  "<CAN3_Rr_RegenAvailTq>"
  RrRegenAvailTq/1(VHAL_RrRegenAvailTq_Nm) -> VHAL_RrRegenAvailTq_Nm/1
  [DT_CAN3_SG_MCU_B_R1] -> bus_selector20/1
  bus_selector20/1 -> RrTMSpd/1(Rr_TMSpd)  "<CAN3_Rr_TMSpd>"
  RrTMSpd/1(VHAL_RrTMSpd_rpm) -> VHAL_RrTMSpd_rpm/1
  [DT_CAN3_SG_MCU_B_R1] -> bus_selector21/1
  bus_selector21/1 -> RrTMTemp/1(Rr_TMTemp)  "<CAN3_Rr_TMTemp>"
  RrTMTemp/1(VHAL_RrTMTemp_C) -> VHAL_RrTMTemp_C/1
  [DT_CAN3_SG_MCU_B_R1] -> bus_selector22/1
  bus_selector22/1 -> RrTMid/1(Rr_TMid)  "<CAN3_Rr_TMid>"
  RrTMid/1(VHAL_RrTMid_A) -> VHAL_RrTMid_A/1
  [DT_CAN3_SG_MCU_B_R1] -> bus_selector23/1
  bus_selector23/1 -> RrTMiq/1(Rr_TMiq)  "<CAN3_Rr_TMiq>"
  RrTMiq/1(VHAL_RrTMiq_A) -> VHAL_RrTMiq_A/1

== system halin/HAL_IN/CAN3/MCU_B_R2 ==
  DT_CAN3_SG_MCU_B_R2 : Inport
  MCUBRLLCTempWarnSta : Subsystem
  RrCoolanttempReq : Subsystem
  RrFailcode1 : Subsystem
  RrFailcode2 : Subsystem
  RrFailcodehistory1 : Subsystem
  RrFailcodehistory2 : Subsystem
  RrLLCTemp : Subsystem
  RrLLCflowReq : Subsystem
  RrMCU3HWVer : Subsystem
  RrMCU3SWVer : Subsystem
  RrMCUTempWarn : Subsystem
  RrTMTempWarn : Subsystem
  bus_selector : BusSelector  OutputSignals=CAN3_MCU_B_R_LLCTempWarn_Sta
  bus_selector1 : BusSelector  OutputSignals=CAN3_Rr_CoolanttempReq
  bus_selector10 : BusSelector  OutputSignals=CAN3_Rr_MCUTempWarn
  bus_selector11 : BusSelector  OutputSignals=CAN3_Rr_TMTempWarn
  bus_selector2 : BusSelector  OutputSignals=CAN3_Rr_Failcode1
  bus_selector3 : BusSelector  OutputSignals=CAN3_Rr_Failcode2
  bus_selector4 : BusSelector  OutputSignals=CAN3_Rr_Failcodehistory1
  bus_selector5 : BusSelector  OutputSignals=CAN3_Rr_Failcodehistory2
  bus_selector6 : BusSelector  OutputSignals=CAN3_Rr_LLCTemp
  bus_selector7 : BusSelector  OutputSignals=CAN3_Rr_LLCflowReq
  bus_selector8 : BusSelector  OutputSignals=CAN3_Rr_MCU3_HW_Ver
  bus_selector9 : BusSelector  OutputSignals=CAN3_Rr_MCU3_SW_Ver
  VHAL_MCUBRLLCTempWarnSta_enum : Outport
  VHAL_RrCoolanttempReq_cnt : Outport  Port=2
  VHAL_RrFailcode1_enum : Outport  Port=3
  VHAL_RrFailcode2_enum : Outport  Port=4
  VHAL_RrFailcodehistory1_enum : Outport  Port=5
  VHAL_RrFailcodehistory2_enum : Outport  Port=6
  VHAL_RrLLCTemp_C : Outport  Port=7
  VHAL_RrLLCflowReq_Lpmin : Outport  Port=8
  VHAL_RrMCU3HWVer_enum : Outport  Port=9
  VHAL_RrMCU3SWVer_enum : Outport  Port=10
  VHAL_RrMCUTempWarn_enum : Outport  Port=11
  VHAL_RrTMTempWarn_enum : Outport  Port=12
  wires:
  DT_CAN3_SG_MCU_B_R2/1 -> [DT_CAN3_SG_MCU_B_R2]
  [DT_CAN3_SG_MCU_B_R2] -> bus_selector/1
  bus_selector/1 -> MCUBRLLCTempWarnSta/1(MCU_B_R_LLCTempWarn_Sta)  "<CAN3_MCU_B_R_LLCTempWarn_Sta>"
  MCUBRLLCTempWarnSta/1(VHAL_MCUBRLLCTempWarnSta_enum) -> VHAL_MCUBRLLCTempWarnSta_enum/1
  [DT_CAN3_SG_MCU_B_R2] -> bus_selector1/1
  bus_selector1/1 -> RrCoolanttempReq/1(Rr_CoolanttempReq)  "<CAN3_Rr_CoolanttempReq>"
  RrCoolanttempReq/1(VHAL_RrCoolanttempReq_cnt) -> VHAL_RrCoolanttempReq_cnt/1
  [DT_CAN3_SG_MCU_B_R2] -> bus_selector2/1
  bus_selector2/1 -> RrFailcode1/1(Rr_Failcode1)  "<CAN3_Rr_Failcode1>"
  RrFailcode1/1(VHAL_RrFailcode1_enum) -> VHAL_RrFailcode1_enum/1
  [DT_CAN3_SG_MCU_B_R2] -> bus_selector3/1
  bus_selector3/1 -> RrFailcode2/1(Rr_Failcode2)  "<CAN3_Rr_Failcode2>"
  RrFailcode2/1(VHAL_RrFailcode2_enum) -> VHAL_RrFailcode2_enum/1
  [DT_CAN3_SG_MCU_B_R2] -> bus_selector4/1
  bus_selector4/1 -> RrFailcodehistory1/1(Rr_Failcodehistory1)  "<CAN3_Rr_Failcodehistory1>"
  RrFailcodehistory1/1(VHAL_RrFailcodehistory1_enum) -> VHAL_RrFailcodehistory1_enum/1
  [DT_CAN3_SG_MCU_B_R2] -> bus_selector5/1
  bus_selector5/1 -> RrFailcodehistory2/1(Rr_Failcodehistory2)  "<CAN3_Rr_Failcodehistory2>"
  RrFailcodehistory2/1(VHAL_RrFailcodehistory2_enum) -> VHAL_RrFailcodehistory2_enum/1
  [DT_CAN3_SG_MCU_B_R2] -> bus_selector6/1
  bus_selector6/1 -> RrLLCTemp/1(Rr_LLCTemp)  "<CAN3_Rr_LLCTemp>"
  RrLLCTemp/1(VHAL_RrLLCTemp_C) -> VHAL_RrLLCTemp_C/1
  [DT_CAN3_SG_MCU_B_R2] -> bus_selector7/1
  bus_selector7/1 -> RrLLCflowReq/1(Rr_LLCflowReq)  "<CAN3_Rr_LLCflowReq>"
  RrLLCflowReq/1(VHAL_RrLLCflowReq_Lpmin) -> VHAL_RrLLCflowReq_Lpmin/1
  [DT_CAN3_SG_MCU_B_R2] -> bus_selector8/1
  bus_selector8/1 -> RrMCU3HWVer/1(Rr_MCU3_HW_Ver)  "<CAN3_Rr_MCU3_HW_Ver>"
  RrMCU3HWVer/1(VHAL_RrMCU3HWVer_enum) -> VHAL_RrMCU3HWVer_enum/1
  [DT_CAN3_SG_MCU_B_R2] -> bus_selector9/1
  bus_selector9/1 -> RrMCU3SWVer/1(Rr_MCU3_SW_Ver)  "<CAN3_Rr_MCU3_SW_Ver>"
  RrMCU3SWVer/1(VHAL_RrMCU3SWVer_enum) -> VHAL_RrMCU3SWVer_enum/1
  [DT_CAN3_SG_MCU_B_R2] -> bus_selector10/1
  bus_selector10/1 -> RrMCUTempWarn/1(Rr_MCUTempWarn)  "<CAN3_Rr_MCUTempWarn>"
  RrMCUTempWarn/1(VHAL_RrMCUTempWarn_enum) -> VHAL_RrMCUTempWarn_enum/1
  [DT_CAN3_SG_MCU_B_R2] -> bus_selector11/1
  bus_selector11/1 -> RrTMTempWarn/1(Rr_TMTempWarn)  "<CAN3_Rr_TMTempWarn>"
  RrTMTempWarn/1(VHAL_RrTMTempWarn_enum) -> VHAL_RrTMTempWarn_enum/1
